simulink model "regPIDnielin"  (R2018b)
settings: Solver=VariableStepAuto  StartTime=0.0  StopTime=10000  RelTol=1e-3
model workspace (MATLAB code in the model file):
  | %classPID(K, Ti, Kd, Td, Tp, Hlim, Llim, Dir, ManVal)
  | 
  | %wpisanie danych
  | C=0.4;
  | a=8;
  | TCp=21;
  | THp=64;
  | TDp=30;
  | FCp=32;
  | FHp=20;
  | FDp=9;
  | tau=40;
  | tau_C=100;
  | hp=58.14;
  | Tp=36.43;
  | Ts = 0.1;
  | 
  | 
  | Ts = 1;
  | Kp1 = 0.600392409469819;
  | Ki1 = 38.51337172496948;
  | 
  | Kp2 = 0.180678962603669;
  | Ki2 = 936.950914688;
  | 
  | global reg1;
  | global reg2;
  | reg1=classPID(Kp1, Ki1, 0, 30, Ts, 50, 0, 1, 1);
  | reg2=classPID(Kp2, Ki2, 0, 30, Ts, 50, 0, 1, 1);
  | 
  | %SetAutoMan(obj, AutoMan, ManVal)
  | reg1.SetAutoMan(1,1);
  | reg2.SetAutoMan(1,1);
settings Model: Creator=Barteux  LastModifiedBy=269823
settings SFSimCC: SimUseLocalCustomCode=off
settings RTWCC: RTWUseLocalCustomCode=off
settings CodeAppCC: StateflowObjectComments=on

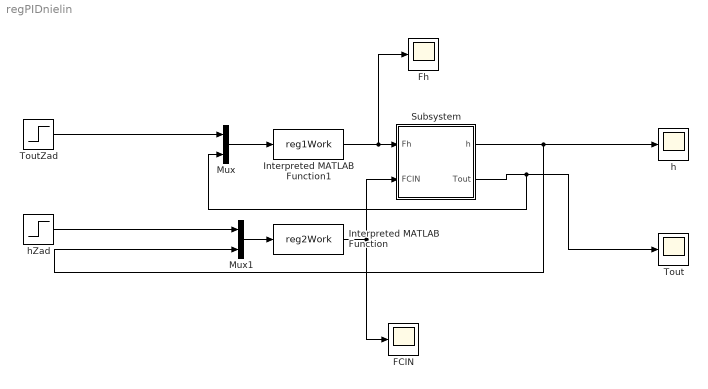
== system regPIDnielin ==
  FCIN : Scope
  "Fh " : Scope
  Interpreted MATLAB Function : MATLABFcn  MATLABFcn=reg2Work  OutputDimensions=1  OutputSignalType=real
  Interpreted MATLAB Function1 : MATLABFcn  MATLABFcn=reg1Work  OutputDimensions=1  OutputSignalType=real
  Mux : Mux  Inputs=2
  Mux1 : Mux  Inputs=2
  Subsystem : Subsystem
  Tout : Scope
  ToutZad : Step  Time=6000  Before=Tp  After=Tp+5  SampleTime=0
  h : Scope
  hZad : Step  Time=3500  Before=hp  After=hp+5  SampleTime=0
  wires:
  Subsystem/1(h) -> Mux1/2, h/1
  Interpreted MATLAB Function/1 -> Subsystem/2(FCIN), FCIN/1
  Mux1/1 -> Interpreted MATLAB Function/1
  hZad/1 -> Mux1/1
  Mux/1 -> Interpreted MATLAB Function1/1
  ToutZad/1 -> Mux/1
  Subsystem/2(Tout) -> Mux/2, Tout/1
  Interpreted MATLAB Function1/1 -> "Fh "/1, Subsystem/1(Fh)

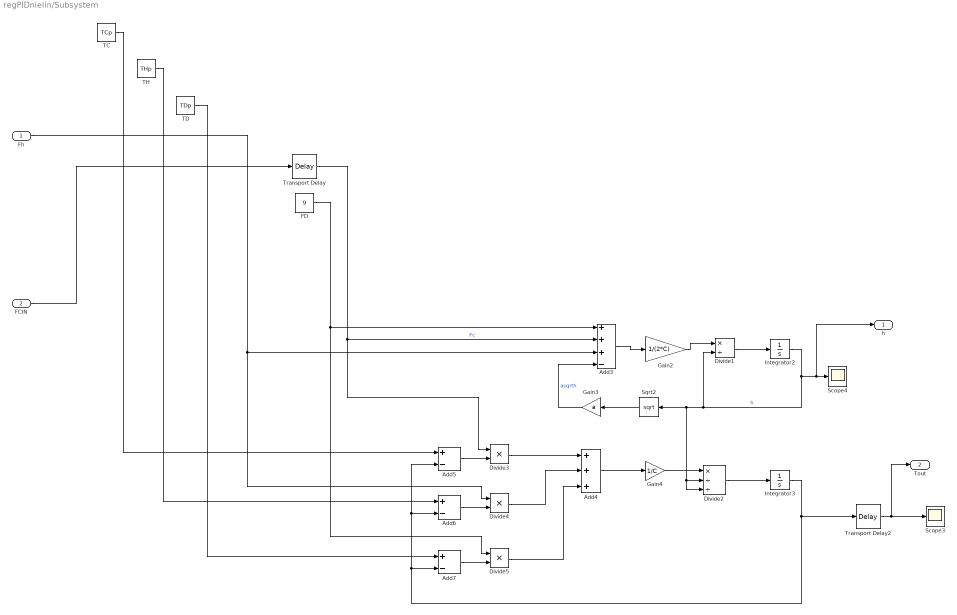
== system regPIDnielin/Subsystem ==
  Fh : Inport
  FCIN : Inport  Port=2
  Add3 : Sum  Inputs=+++-
  Add4 : Sum  Inputs=+++
  Add5 : Sum  Inputs=+-
  Add6 : Sum  Inputs=+-
  Add7 : Sum  Inputs=+-
  Divide1 : Product  Inputs=*/
  Divide2 : Product  Inputs=*//
  Divide3 : Product  Inputs=**
  Divide4 : Product  Inputs=**
  Divide5 : Product  Inputs=**
  FD : Constant  Value=9
  Gain2 : Gain  Gain=1/(2*C)
  Gain3 : Gain  Gain=a
  Gain4 : Gain  Gain=1/C
  Integrator2 : Integrator  InitialCondition=hp
  Integrator3 : Integrator  InitialCondition=Tp
  Scope3 : Scope
  Scope4 : Scope
  Sqrt2 : Sqrt  OutputSignalType=real  SaturateOnIntegerOverflow=on
  TC : Constant  Value=TCp
  TD : Constant  Value=TDp
  TH : Constant  Value=THp
  Transport Delay : TransportDelay  DelayTime=tau_C
  Transport Delay2 : TransportDelay  DelayTime=tau
  h : Outport
  Tout : Outport  Port=2
  wires:
  Fh/1 -> Divide4/1, Add3/3
  TD/1 -> Add7/1
  TH/1 -> Add6/1
  Transport Delay/1 -> Divide3/1, Add3/2  "Fc"
  FD/1 -> Divide5/1, Add3/1
  Integrator2/1 -> h/1, Scope4/1, Divide2/3, Divide2/2, Sqrt2/1, Divide1/2  "h"
  Add5/1 -> Divide3/2
  Sqrt2/1 -> Gain3/1
  Gain4/1 -> Divide2/1
  Divide1/1 -> Integrator2/1
  Add3/1 -> Gain2/1
  Divide2/1 -> Integrator3/1
  Add6/1 -> Divide4/2
  Add4/1 -> Gain4/1
  Gain2/1 -> Divide1/1
  Transport Delay2/1 -> Tout/1, Scope3/1
  Gain3/1 -> Add3/4  "asqrth"
  Divide5/1 -> Add4/3
  TC/1 -> Add5/1
  Integrator3/1 -> Add7/2, Add6/2, Add5/2, Transport Delay2/1
  Divide3/1 -> Add4/1
  Add7/1 -> Divide5/2
  Divide4/1 -> Add4/2
  FCIN/1 -> Transport Delay/1
